simulink model "AutopilotControlSystem"  (R2019b)
settings: configuration reference "ctrlConfigSet" (kept outside this file)
undefined symbols (not defined in the file): ap, DiscIntNeverNeededParam, Earth, env, sensors, uav, WGS84
libraries: mbdriLib x74, simulink x12, aerolibtransform2 x5, simulink_need_slupdate x1, aerolibconvert2 x1
(part 1 of 3)
settings Model: ParamWorkspaceSource=ReferencedWorkspace  Creator=mlizarra  LastModifiedBy=ben
settings ConfigSetRef: SourceName=ctrlConfigSet  SourceLocation=Base Workspace

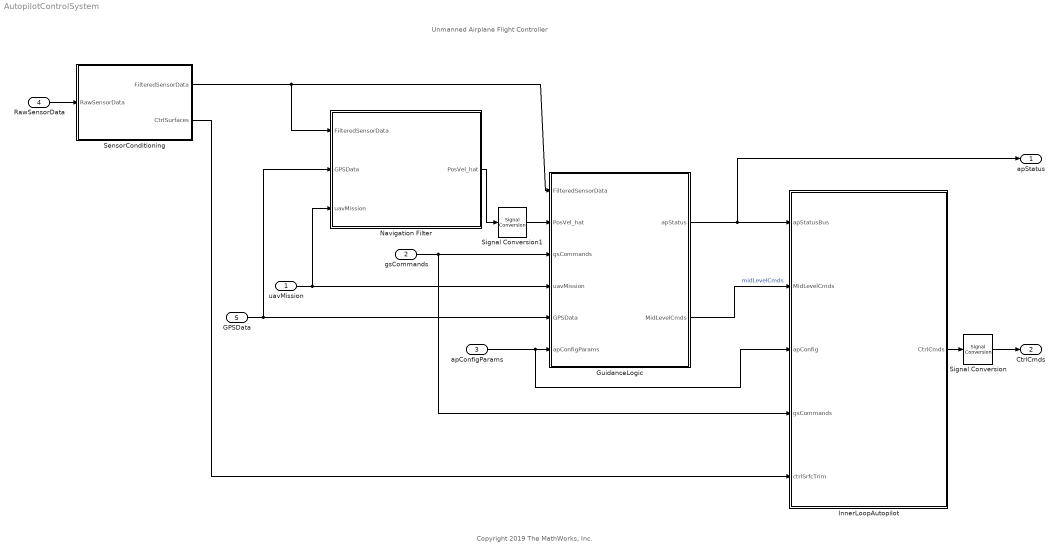
== system AutopilotControlSystem ==
  note: Copyright 2019 The MathWorks, Inc.
  note: Unmanned Airplane Flight Controller
  uavMission : Inport  OutDataTypeStr=Bus: waypoint  PortDimensions=10  SampleTime=[0.01,0]  BusOutputAsStruct=on
  gsCommands : Inport  Port=2  OutDataTypeStr=Bus: gsCommandsBus  PortDimensions=1  SampleTime=[0.01,0]  BusOutputAsStruct=on
  apConfigParams : Inport  Port=3  OutDataTypeStr=Bus: apConfigParamsBus  PortDimensions=1  SampleTime=[0.01,0]  BusOutputAsStruct=on
  RawSensorData : Inport  Port=4  OutDataTypeStr=Bus: rawSensorDataBus  PortDimensions=1  SampleTime=[0.01,0]  BusOutputAsStruct=on
  GPSData : Inport  Port=5  OutDataTypeStr=Bus: gpsReading  PortDimensions=1  SampleTime=[0.01,0]  BusOutputAsStruct=on
  GuidanceLogic : Subsystem  Variant=on  VariantControl=Variant1
  InnerLoopAutopilot : Subsystem  TreatAsAtomicUnit=on
  Navigation Filter : Subsystem  TreatAsAtomicUnit=on
  SensorConditioning : Subsystem  TreatAsAtomicUnit=on
  Signal Conversion : SignalConversion  ConversionOutput=Nonvirtual bus  OutDataTypeStr=Bus: ctrlCmdsBus  OverrideOpt=off
  Signal Conversion1 : SignalConversion  ConversionOutput=Nonvirtual bus  OutDataTypeStr=Bus: PosVel_hat  OverrideOpt=off
  apStatus : Outport  OutDataTypeStr=Bus: apStatusBus  PortDimensions=1  SampleTime=[0.01,0]  VectorParamsAs1DForOutWhenUnconnected=off  BusOutputAsStruct=on
  CtrlCmds : Outport  Port=2  OutDataTypeStr=Bus: ctrlCmdsBus  SampleTime=[0.01,0]  VectorParamsAs1DForOutWhenUnconnected=off  BusOutputAsStruct=on
  wires:
  gsCommands/1 -> GuidanceLogic/3("gsCommands "), InnerLoopAutopilot/4(gsCommands)
  uavMission/1 -> Navigation Filter/3(uavMission), GuidanceLogic/4("uavMission ")
  GuidanceLogic/2(" MidLevelCmds") -> InnerLoopAutopilot/2(MidLevelCmds)  "midLevelCmds"
  Navigation Filter/1(PosVel_hat) -> Signal Conversion1/1
  GPSData/1 -> Navigation Filter/2(GPSData), GuidanceLogic/5("GPSData ")
  SensorConditioning/2(CtrlSurfaces) -> InnerLoopAutopilot/5(ctrlSrfcTrim)
  SensorConditioning/1(FilteredSensorData) -> Navigation Filter/1(FilteredSensorData), GuidanceLogic/1("FilteredSensorData ")
  GuidanceLogic/1(" apStatus") -> InnerLoopAutopilot/1(apStatusBus), apStatus/1
  apConfigParams/1 -> InnerLoopAutopilot/3(apConfig), GuidanceLogic/6("apConfigParams ")
  RawSensorData/1 -> SensorConditioning/1(RawSensorData)
  InnerLoopAutopilot/1(CtrlCmds) -> Signal Conversion/1
  Signal Conversion/1 -> CtrlCmds/1
  Signal Conversion1/1 -> GuidanceLogic/2("PosVel_hat ")

== system AutopilotControlSystem/GuidanceLogic ==
  "FilteredSensorData " : Inport
  "PosVel_hat " : Inport  Port=2
  "gsCommands " : Inport  Port=3
  "uavMission " : Inport  Port=4
  "GPSData " : Inport  Port=5
  "apConfigParams " : Inport  Port=6
  GuidanceLogic_Simulink : Subsystem  TreatAsAtomicUnit=on  VariantControl=useSLguidance
  GuidanceLogic_Stateflow : Subsystem  TreatAsAtomicUnit=on  VariantControl=useSFguidance
  " apStatus" : Outport  VectorParamsAs1DForOutWhenUnconnected=off
  " MidLevelCmds" : Outport  Port=2  VectorParamsAs1DForOutWhenUnconnected=off

== system AutopilotControlSystem/InnerLoopAutopilot ==
  apStatusBus : Inport  OutDataTypeStr=Bus: apStatusBus
  MidLevelCmds : Inport  Port=2
  apConfig : Inport  Port=3  OutDataTypeStr=Bus: apConfigParamsBus
  gsCommands : Inport  Port=4
  ctrlSrfcTrim : Inport  Port=5
  FLapCmd : Constant  Value=0  OutDataTypeStr=single  SampleTime=ap.apSampleTime
      settings: AttributesFormatString=%<Value>
  Latch Trim Conditions : Subsystem
  Lateral Channel : Subsystem  TreatAsAtomicUnit=on
  Longitudinal Channel : Subsystem  TreatAsAtomicUnit=on
  Out Bus Element : Outport  VectorParamsAs1DForOutWhenUnconnected=off  PortName=CtrlCmds  Element=elevatorCmd
  Out Bus Element1 : Outport  VectorParamsAs1DForOutWhenUnconnected=off  PortName=CtrlCmds  Element=throttleCmd
  Out Bus Element2 : Outport  VectorParamsAs1DForOutWhenUnconnected=off  PortName=CtrlCmds  Element=aileronCmd
  Out Bus Element3 : Outport  VectorParamsAs1DForOutWhenUnconnected=off  PortName=CtrlCmds  Element=rudderCmd
  Out Bus Element4 : Outport  VectorParamsAs1DForOutWhenUnconnected=off  PortName=CtrlCmds  Element=flapCmd
  wires:
  gsCommands/1 -> Latch Trim Conditions/2(gsCommands), Lateral Channel/5(gsCommands), Longitudinal Channel/5(gsCommands)
  Latch Trim Conditions/1(CtrlSrfcTrim) -> Lateral Channel/4(ctrlSrfcTrim), Longitudinal Channel/4(ctrlSrfcTrim)
  ctrlSrfcTrim/1 -> Latch Trim Conditions/1(ctrlSurfaces)
  apConfig/1 -> Lateral Channel/3(apConfigBus), Longitudinal Channel/3(apConfigBus)
  FLapCmd/1 -> Out Bus Element4/1
  Lateral Channel/2(dR) -> Out Bus Element3/1
  Lateral Channel/1(dA) -> Out Bus Element2/1
  Longitudinal Channel/2(dT) -> Out Bus Element1/1
  Longitudinal Channel/1(dE) -> Out Bus Element/1
  apStatusBus/1 -> Lateral Channel/2(apStatusBus), Longitudinal Channel/2(apStatusBus)
  MidLevelCmds/1 -> Lateral Channel/1(midLevelCmds), Longitudinal Channel/1(midLevelCmds)

== system AutopilotControlSystem/Navigation Filter ==
  In Bus Element5 : Inport  PortName=FilteredSensorData  Element=Euler
  In Bus Element6 : Inport  PortName=FilteredSensorData  Element=Ab
  In Bus Element7 : Inport  PortName=FilteredSensorData  Element=baro
  In Bus Element : Inport  Port=2  PortName=GPSData  Element=gps_fix
  In Bus Element1 : Inport  Port=2  PortName=GPSData  Element=gps_latLon
  In Bus Element2 : Inport  Port=2  PortName=GPSData  Element=gps_h
  In Bus Element3 : Inport  Port=2  PortName=GPSData  Element=gps_cog
  In Bus Element4 : Inport  Port=2  PortName=GPSData  Element=gps_sog
  uavMission : Inport  Port=3  OutDataTypeStr=Bus: waypoint
  Baro Altimeter : Subsystem
  Bus Selector1 : BusSelector  OutputSignals=wpPos
  Compare To Constant : simulink/Logic and Bit Operations/Compare To Constant  relop=>=  const=3  OutDataTypeStr=boolean
  GPS Update : Subsystem  mask{T=ap.apSampleTime}
      mask prompts: T "Sample Time"
  Get Vn Ve : Subsystem
  LLA to Flat Earth : Subsystem
  Position&Velocity Filter : Subsystem
  RL2B : mbdriLib/Coordinates/RL2B  SystemSampleTime=-1  Latency=0  AutoFrameSizeCalculation=off
      settings: SourceProductName=Robotics System Toolbox  SourceProductBaseCode=RO
  Selector : Selector  InputPortWidth=10  IndexOptions=Index vector (dialog)  Indices=[1]  OutputSizes=1
  get Height : Selector  InputPortWidth=3  IndexOptions=Index vector (dialog)  Indices=[3]  OutputSizes=1
  Out Bus Element : Outport  VectorParamsAs1DForOutWhenUnconnected=off  PortName=PosVel_hat  Element=Ve_hat
  Out Bus Element1 : Outport  VectorParamsAs1DForOutWhenUnconnected=off  PortName=PosVel_hat  Element=Xe_hat
  Out Bus Element2 : Outport  VectorParamsAs1DForOutWhenUnconnected=off  PortName=PosVel_hat  Element=Ab_bias_hat
  wires:
  LLA to Flat Earth/1(Xe) -> Position&Velocity Filter/2(Xe), GPS Update/1(Xe)
  get Height/1 -> Position&Velocity Filter/9(Base Height)
  In Bus Element6/1 -> Position&Velocity Filter/7(A_sens)
  RL2B/1 -> Position&Velocity Filter/6(RLT2B)
  In Bus Element5/1 -> RL2B/1
  In Bus Element7/1 -> Baro Altimeter/1(Static (Pa))
  Baro Altimeter/1(Altitude) -> Position&Velocity Filter/8(BaroAlt)
  Get Vn Ve/2(Veast) -> Position&Velocity Filter/4(Veast)
  Get Vn Ve/1(Vnorth) -> Position&Velocity Filter/3(Vnorth)
  GPS Update/1(Update?) -> Position&Velocity Filter/1(NewGPS)
  Selector/1 -> Bus Selector1/1
  uavMission/1 -> Selector/1
  Bus Selector1/1 -> LLA to Flat Earth/5(initPos), get Height/1  "<wpPos>"
  In Bus Element4/1 -> LLA to Flat Earth/4(SOG)
  In Bus Element3/1 -> LLA to Flat Earth/3(COG)
  In Bus Element2/1 -> LLA to Flat Earth/2(h)
  In Bus Element1/1 -> LLA to Flat Earth/1(latLon)
  Compare To Constant/1 -> LLA to Flat Earth/Enable
  In Bus Element/1 -> Compare To Constant/1
  Position&Velocity Filter/2(Xe_hat) -> Out Bus Element1/1
  Position&Velocity Filter/1(Ve_hat) -> Out Bus Element/1
  Position&Velocity Filter/3(acc_bias) -> Out Bus Element2/1
  LLA to Flat Earth/2(COG_out) -> Get Vn Ve/1(COG)
  LLA to Flat Earth/3(SOG_out) -> Get Vn Ve/2(SOG), Position&Velocity Filter/5(SOG)

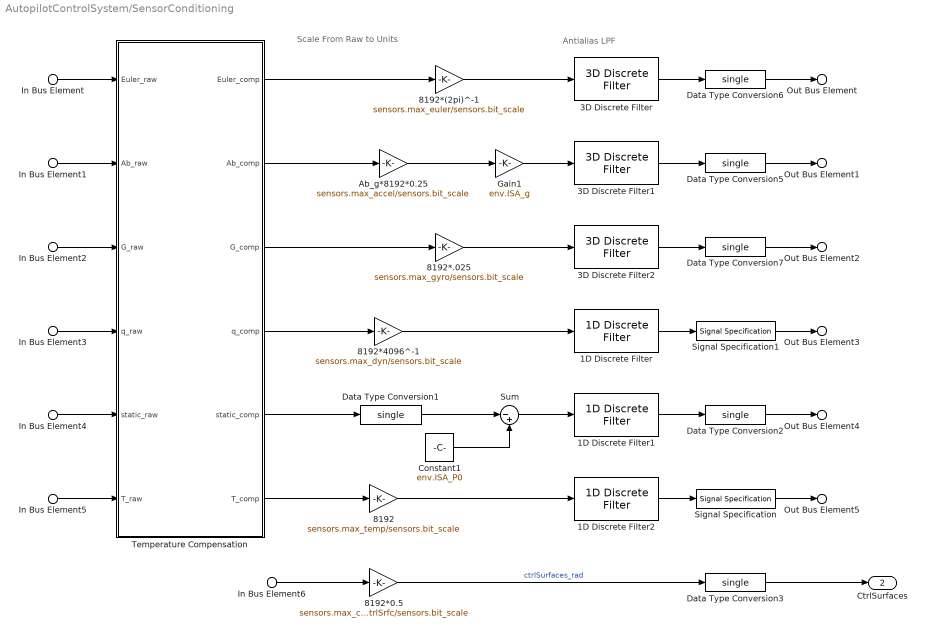
== system AutopilotControlSystem/SensorConditioning ==
  note: Antialias LPF
  note: Scale From Raw to Units
  In Bus Element : Inport  PortName=RawSensorData  Element=Euler_raw
  In Bus Element1 : Inport  PortName=RawSensorData  Element=Ab_raw
  In Bus Element2 : Inport  PortName=RawSensorData  Element=G_raw
  In Bus Element3 : Inport  PortName=RawSensorData  Element=q_raw
  In Bus Element4 : Inport  PortName=RawSensorData  Element=static_raw
  In Bus Element5 : Inport  PortName=RawSensorData  Element=T_raw
  In Bus Element6 : Inport  PortName=RawSensorData  Element=ctrlSurface_PWM
  1D Discrete Filter : mbdriLib/Filtering/1D Discrete Filter  bw=sensors.antialiasBW  TSample=ap.apSampleTime
      settings: AttributesFormatString=Fc = 40  SourceProductName=Robotics System Toolbox  SourceProductBaseCode=RO
  1D Discrete Filter1 : mbdriLib/Filtering/1D Discrete Filter  bw=sensors.antialiasBW  TSample=ap.apSampleTime
      settings: AttributesFormatString=Fc = 40  SourceProductName=Robotics System Toolbox  SourceProductBaseCode=RO
  1D Discrete Filter2 : mbdriLib/Filtering/1D Discrete Filter  bw=sensors.antialiasBW  TSample=ap.apSampleTime
      settings: AttributesFormatString=Fc = 40  SourceProductName=Robotics System Toolbox  SourceProductBaseCode=RO
  3D Discrete Filter : mbdriLib/Filtering/3D Discrete Filter  bw=sensors.antialiasBW  TSample=ap.apSampleTime
      settings: AttributesFormatString=Fc = 40  SourceProductName=Robotics System Toolbox  SourceProductBaseCode=RO
  3D Discrete Filter1 : mbdriLib/Filtering/3D Discrete Filter  bw=sensors.antialiasBW  TSample=ap.apSampleTime
      settings: AttributesFormatString=Fc = 40  SourceProductName=Robotics System Toolbox  SourceProductBaseCode=RO
  3D Discrete Filter2 : mbdriLib/Filtering/3D Discrete Filter  bw=sensors.antialiasBW  TSample=ap.apSampleTime
      settings: AttributesFormatString=Fc = 40  SourceProductName=Robotics System Toolbox  SourceProductBaseCode=RO
  8192 : Gain  Description=8192/1  Gain=sensors.max_temp/sensors.bit_scale  OutDataTypeStr=single
      settings: AttributesFormatString=%<Gain>
  8192*(2pi)^-1 : Gain  Gain=sensors.max_euler/sensors.bit_scale  OutDataTypeStr=single
      settings: AttributesFormatString=%<Gain>
  8192*.025 : Gain  Gain=sensors.max_gyro/sensors.bit_scale  OutDataTypeStr=single
      settings: AttributesFormatString=%<Gain>
  8192*0.5 : Gain  Gain=sensors.max_ctrlSrfc/sensors.bit_scale  OutDataTypeStr=single
      settings: AttributesFormatString=%<Gain>
  8192*4096^-1 : Gain  Gain=sensors.max_dyn/sensors.bit_scale  OutDataTypeStr=single
      settings: AttributesFormatString=%<Gain>
  Ab_g*8192*0.25 : Gain  Gain=sensors.max_accel/sensors.bit_scale  OutDataTypeStr=single
      settings: AttributesFormatString=%<Gain>
  Constant1 : Constant  Value=env.ISA_P0
      settings: AttributesFormatString=%<Value>
  Data Type Conversion{1..3,5..7} (6 alike) : DataTypeConversion  OutDataTypeStr=single
  Gain1 : Gain  Gain=env.ISA_g  OutDataTypeStr=single
      settings: AttributesFormatString=%<Gain>
  Signal Specification : SignalSpecification  OutDataTypeStr=single  Unit=K
  Signal Specification1 : SignalSpecification  OutDataTypeStr=single  Unit=Pa
  Sum : Sum  Inputs=|-+
  Temperature Compensation : Subsystem
  Out Bus Element : Outport  VectorParamsAs1DForOutWhenUnconnected=off  PortName=FilteredSensorData  Element=Euler
  Out Bus Element1 : Outport  VectorParamsAs1DForOutWhenUnconnected=off  PortName=FilteredSensorData  Element=Ab
  Out Bus Element2 : Outport  VectorParamsAs1DForOutWhenUnconnected=off  PortName=FilteredSensorData  Element=G
  Out Bus Element3 : Outport  VectorParamsAs1DForOutWhenUnconnected=off  PortName=FilteredSensorData  Element=q
  Out Bus Element4 : Outport  VectorParamsAs1DForOutWhenUnconnected=off  PortName=FilteredSensorData  Element=baro
  Out Bus Element5 : Outport  VectorParamsAs1DForOutWhenUnconnected=off  PortName=FilteredSensorData  Element=T
  CtrlSurfaces : Outport  Port=2  VectorParamsAs1DForOutWhenUnconnected=off
  wires:
  8192*0.5/1 -> Data Type Conversion3/1  "ctrlSurfaces_rad"
  In Bus Element6/1 -> 8192*0.5/1
  Data Type Conversion3/1 -> CtrlSurfaces/1
  1D Discrete Filter2/1 -> Signal Specification/1
  Data Type Conversion2/1 -> Out Bus Element4/1
  1D Discrete Filter1/1 -> Data Type Conversion2/1
  1D Discrete Filter/1 -> Signal Specification1/1
  3D Discrete Filter2/1 -> Data Type Conversion7/1
  3D Discrete Filter1/1 -> Data Type Conversion5/1
  3D Discrete Filter/1 -> Data Type Conversion6/1
  Data Type Conversion1/1 -> Sum/1
  Gain1/1 -> 3D Discrete Filter1/1
  Data Type Conversion6/1 -> Out Bus Element/1
  Data Type Conversion5/1 -> Out Bus Element1/1
  Data Type Conversion7/1 -> Out Bus Element2/1
  Signal Specification1/1 -> Out Bus Element3/1
  Sum/1 -> 1D Discrete Filter1/1
  Signal Specification/1 -> Out Bus Element5/1
  Constant1/1 -> Sum/2
  8192/1 -> 1D Discrete Filter2/1
  8192*4096^-1/1 -> 1D Discrete Filter/1
  8192*.025/1 -> 3D Discrete Filter2/1
  8192*(2pi)^-1/1 -> 3D Discrete Filter/1
  Ab_g*8192*0.25/1 -> Gain1/1
  In Bus Element/1 -> Temperature Compensation/1(Euler_raw)
  In Bus Element1/1 -> Temperature Compensation/2(Ab_raw)
  In Bus Element2/1 -> Temperature Compensation/3(G_raw)
  In Bus Element3/1 -> Temperature Compensation/4(q_raw)
  In Bus Element4/1 -> Temperature Compensation/5(static_raw)
  In Bus Element5/1 -> Temperature Compensation/6(T_raw)
  Temperature Compensation/1(Euler_comp) -> 8192*(2pi)^-1/1
  Temperature Compensation/2(Ab_comp) -> Ab_g*8192*0.25/1
  Temperature Compensation/3(G_comp) -> 8192*.025/1
  Temperature Compensation/4(q_comp) -> 8192*4096^-1/1
  Temperature Compensation/5(static_comp) -> Data Type Conversion1/1
  Temperature Compensation/6(T_comp) -> 8192/1

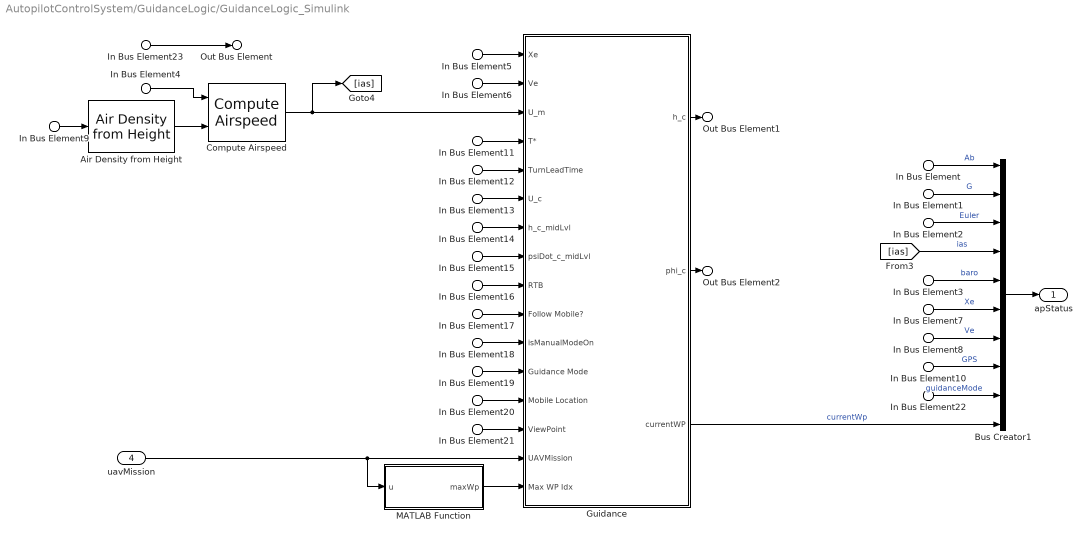
== system AutopilotControlSystem/GuidanceLogic/GuidanceLogic_Simulink ==
  In Bus Element : Inport  PortName=FilteredSensorData  Element=Ab
  In Bus Element1 : Inport  PortName=FilteredSensorData  Element=G
  In Bus Element2 : Inport  PortName=FilteredSensorData  Element=Euler
  In Bus Element3 : Inport  PortName=FilteredSensorData  Element=baro
  In Bus Element4 : Inport  PortName=FilteredSensorData  Element=q
  In Bus Element5 : Inport  Port=2  PortName=PosVel_hat  Element=Xe_hat
  In Bus Element7 : Inport  Port=2  PortName=PosVel_hat  Element=Xe_hat
  In Bus Element6 : Inport  Port=2  PortName=PosVel_hat  Element=Ve_hat
  In Bus Element8 : Inport  Port=2  PortName=PosVel_hat  Element=Ve_hat
  In Bus Element13 : Inport  Port=3  PortName=gsCommands  Element=U_c
  In Bus Element23 : Inport  Port=3  PortName=gsCommands  Element=U_c
  In Bus Element14 : Inport  Port=3  PortName=gsCommands  Element=h_c_midLevel
  In Bus Element15 : Inport  Port=3  PortName=gsCommands  Element=psiDot_c_midLevel
  In Bus Element16 : Inport  Port=3  PortName=gsCommands  Element=RTB
  In Bus Element17 : Inport  Port=3  PortName=gsCommands  Element=followMobile
  In Bus Element18 : Inport  Port=3  PortName=gsCommands  Element=isManualModeOn
  In Bus Element19 : Inport  Port=3  PortName=gsCommands  Element=guidanceMode
  In Bus Element22 : Inport  Port=3  PortName=gsCommands  Element=guidanceMode
  In Bus Element20 : Inport  Port=3  PortName=gsCommands  Element=MobileLocation
  In Bus Element21 : Inport  Port=3  PortName=gsCommands  Element=viewPointIdx
  uavMission : Inport  Port=4
  In Bus Element10 : Inport  Port=5  PortName=GPSData
  In Bus Element9 : Inport  Port=5  PortName=GPSData  Element=gps_h
  In Bus Element11 : Inport  Port=6  PortName=apConfigParams  Element=T_star
  In Bus Element12 : Inport  Port=6  PortName=apConfigParams  Element=turnLead
  Air Density from Height : mbdriLib/Air Utilities/Air Density from Height  SystemSampleTime=-1  Latency=0  AutoFrameSizeCalculation=off
      settings: SourceProductName=Robotics System Toolbox  SourceProductBaseCode=RO
  Bus Creator1 : BusCreator  Inputs=10  OutDataTypeStr=Bus: apStatusBus  NonVirtualBus=on
  Compute Airspeed : mbdriLib/Air Utilities/Compute Airspeed  SystemSampleTime=-1  Latency=0  AutoFrameSizeCalculation=off
      settings: SourceProductName=Robotics System Toolbox  SourceProductBaseCode=RO
  Guidance : Subsystem  TreatAsAtomicUnit=on
  MATLAB Function : MATLAB Function  TreatAsAtomicUnit=on
  apStatus : Outport  VectorParamsAs1DForOutWhenUnconnected=off
  Out Bus Element : Outport  Port=2  VectorParamsAs1DForOutWhenUnconnected=off  PortName=MidLevelCmds  Element=U_c
  Out Bus Element1 : Outport  Port=2  VectorParamsAs1DForOutWhenUnconnected=off  PortName=MidLevelCmds  Element=h_c
  Out Bus Element2 : Outport  Port=2  VectorParamsAs1DForOutWhenUnconnected=off  PortName=MidLevelCmds  Element=phi_c
  wires:
  Guidance/3(currentWP) -> Bus Creator1/10  "currentWp"
  In Bus Element22/1 -> Bus Creator1/9  "guidanceMode"
  In Bus Element10/1 -> Bus Creator1/8  "GPS"
  In Bus Element8/1 -> Bus Creator1/7  "Ve"
  In Bus Element7/1 -> Bus Creator1/6  "Xe"
  In Bus Element3/1 -> Bus Creator1/5  "baro"
  [ias] -> Bus Creator1/4  "ias"
  In Bus Element2/1 -> Bus Creator1/3  "Euler"
  In Bus Element1/1 -> Bus Creator1/2  "G"
  In Bus Element/1 -> Bus Creator1/1  "Ab"
  Bus Creator1/1 -> apStatus/1
  Guidance/2(phi_c) -> Out Bus Element2/1
  Guidance/1(h_c) -> Out Bus Element1/1
  In Bus Element9/1 -> Air Density from Height/1
  In Bus Element12/1 -> Guidance/5(TurnLeadTime)
  In Bus Element11/1 -> Guidance/4("T* ")
  MATLAB Function/1(maxWp) -> Guidance/16(Max WP Idx)
  In Bus Element4/1 -> Compute Airspeed/1
  Compute Airspeed/1 -> Guidance/3(U_m), [ias]
  Air Density from Height/1 -> Compute Airspeed/2
  In Bus Element21/1 -> Guidance/14(ViewPoint)
  In Bus Element20/1 -> Guidance/13(Mobile Location)
  In Bus Element19/1 -> Guidance/12(Guidance Mode)
  In Bus Element18/1 -> Guidance/11(isManualModeOn)
  In Bus Element17/1 -> Guidance/10(Follow Mobile?)
  In Bus Element16/1 -> Guidance/9(RTB)
  In Bus Element15/1 -> Guidance/8(psiDot_c_midLvl)
  In Bus Element14/1 -> Guidance/7(h_c_midLvl)
  In Bus Element13/1 -> Guidance/6(U_c)
  In Bus Element6/1 -> Guidance/2(Ve)
  In Bus Element5/1 -> Guidance/1(Xe)
  uavMission/1 -> Guidance/15(UAVMission), MATLAB Function/1(u)
  In Bus Element23/1 -> Out Bus Element/1

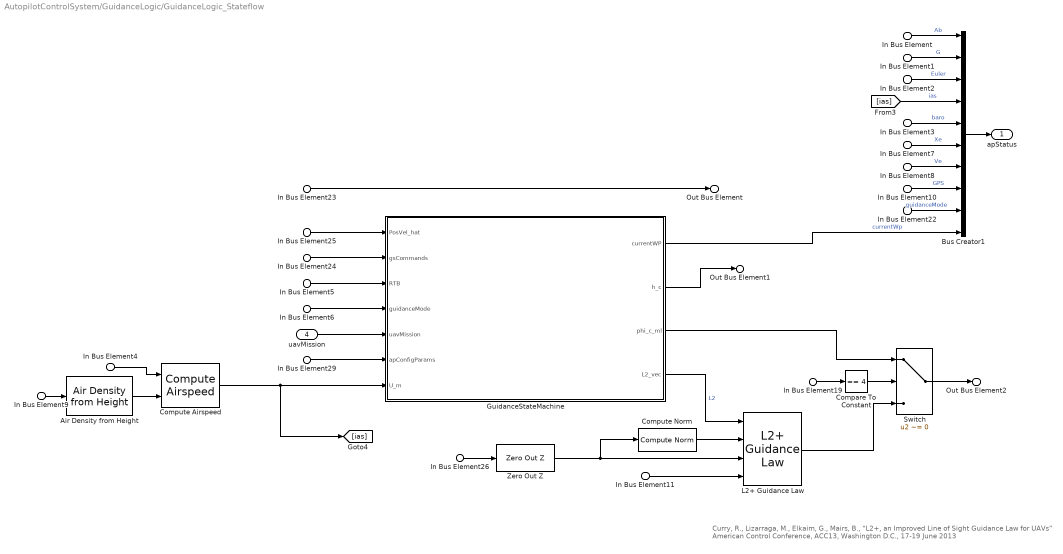
== system AutopilotControlSystem/GuidanceLogic/GuidanceLogic_Stateflow ==
  note: Curry, R., Lizarraga, M., Elkaim, G., Mairs, B., “L2+, an Improved Line of Sight Guidance Law for UAVs”
      | American Control Conference, ACC13, Washington D.C., 17-19 June 2013
  In Bus Element : Inport  PortName=FilteredSensorData  Element=Ab
  In Bus Element1 : Inport  PortName=FilteredSensorData  Element=G
  In Bus Element2 : Inport  PortName=FilteredSensorData  Element=Euler
  In Bus Element3 : Inport  PortName=FilteredSensorData  Element=baro
  In Bus Element4 : Inport  PortName=FilteredSensorData  Element=q
  In Bus Element25 : Inport  Port=2  PortName=PosVel_hat
  In Bus Element7 : Inport  Port=2  PortName=PosVel_hat  Element=Xe_hat
  In Bus Element8 : Inport  Port=2  PortName=PosVel_hat  Element=Ve_hat
  In Bus Element26 : Inport  Port=2  PortName=PosVel_hat  Element=Ve_hat
  In Bus Element24 : Inport  Port=3  PortName=gsCommands
  In Bus Element23 : Inport  Port=3  PortName=gsCommands  Element=U_c
  In Bus Element19 : Inport  Port=3  PortName=gsCommands  Element=guidanceMode
  In Bus Element22 : Inport  Port=3  PortName=gsCommands  Element=guidanceMode
  In Bus Element6 : Inport  Port=3  PortName=gsCommands  Element=guidanceMode
  In Bus Element5 : Inport  Port=3  PortName=gsCommands  Element=RTB
  uavMission : Inport  Port=4
  In Bus Element10 : Inport  Port=5  PortName=GPSData
  In Bus Element9 : Inport  Port=5  PortName=GPSData  Element=gps_h
  In Bus Element29 : Inport  Port=6  PortName=apConfigParams
  In Bus Element11 : Inport  Port=6  PortName=apConfigParams  Element=T_star
  " Compute Norm" : mbdriLib/Utilities/ Compute Norm  SystemSampleTime=-1  Latency=0  AutoFrameSizeCalculation=off
      settings: SourceProductName=Robotics System Toolbox  SourceProductBaseCode=RO
  Air Density from Height : mbdriLib/Air Utilities/Air Density from Height  SystemSampleTime=-1  Latency=0  AutoFrameSizeCalculation=off
      settings: SourceProductName=Robotics System Toolbox  SourceProductBaseCode=RO
  Bus Creator1 : BusCreator  Inputs=10  OutDataTypeStr=Bus: apStatusBus  NonVirtualBus=on
  Compare To Constant : simulink/Logic and Bit Operations/Compare To Constant  relop===  const=4  OutDataTypeStr=boolean
  Compute Airspeed : mbdriLib/Air Utilities/Compute Airspeed  SystemSampleTime=-1  Latency=0  AutoFrameSizeCalculation=off
      settings: SourceProductName=Robotics System Toolbox  SourceProductBaseCode=RO
  GuidanceStateMachine : Stateflow chart  TreatAsAtomicUnit=on
  L2+ Guidance Law : mbdriLib/Guidance/L2+ Guidance Law  SystemSampleTime=-1  Latency=0  AutoFrameSizeCalculation=off
      settings: SourceProductName=Robotics System Toolbox  SourceProductBaseCode=RO
  Switch : Switch  Criteria=u2 ~= 0  Threshold=3.1
  Zero Out Z : mbdriLib/Utilities/Zero Out Z  SystemSampleTime=-1  Latency=0  AutoFrameSizeCalculation=off
      settings: SourceProductName=Robotics System Toolbox  SourceProductBaseCode=RO
  apStatus : Outport  VectorParamsAs1DForOutWhenUnconnected=off
  Out Bus Element : Outport  Port=2  VectorParamsAs1DForOutWhenUnconnected=off  PortName=MidLevelCmds  Element=U_c
  Out Bus Element1 : Outport  Port=2  VectorParamsAs1DForOutWhenUnconnected=off  PortName=MidLevelCmds  Element=h_c
  Out Bus Element2 : Outport  Port=2  VectorParamsAs1DForOutWhenUnconnected=off  PortName=MidLevelCmds  Element=phi_c
  wires:
  In Bus Element23/1 -> Out Bus Element/1
  Air Density from Height/1 -> Compute Airspeed/2
  In Bus Element4/1 -> Compute Airspeed/1
  In Bus Element9/1 -> Air Density from Height/1
  Bus Creator1/1 -> apStatus/1
  In Bus Element/1 -> Bus Creator1/1  "Ab"
  In Bus Element1/1 -> Bus Creator1/2  "G"
  In Bus Element2/1 -> Bus Creator1/3  "Euler"
  [ias] -> Bus Creator1/4  "ias"
  In Bus Element3/1 -> Bus Creator1/5  "baro"
  In Bus Element7/1 -> Bus Creator1/6  "Xe"
  In Bus Element8/1 -> Bus Creator1/7  "Ve"
  In Bus Element10/1 -> Bus Creator1/8  "GPS"
  In Bus Element22/1 -> Bus Creator1/9  "guidanceMode"
  In Bus Element24/1 -> GuidanceStateMachine/2(gsCommands)
  uavMission/1 -> GuidanceStateMachine/5(uavMission)
  In Bus Element25/1 -> GuidanceStateMachine/1(PosVel_hat)
  In Bus Element29/1 -> GuidanceStateMachine/6(apConfigParams)
  Compute Airspeed/1 -> GuidanceStateMachine/7(U_m), [ias]
  GuidanceStateMachine/1(currentWP) -> Bus Creator1/10  "currentWp"
  GuidanceStateMachine/2(h_c) -> Out Bus Element1/1
  Switch/1 -> Out Bus Element2/1
  " Compute Norm"/1 -> L2+ Guidance Law/2
  GuidanceStateMachine/4(L2_vec) -> L2+ Guidance Law/1  "L2"
  In Bus Element11/1 -> L2+ Guidance Law/4
  Zero Out Z/1 -> L2+ Guidance Law/3, " Compute Norm"/1
  GuidanceStateMachine/3(phi_c_ml) -> Switch/1
  In Bus Element19/1 -> Compare To Constant/1
  L2+ Guidance Law/1 -> Switch/3
  In Bus Element26/1 -> Zero Out Z/1
  In Bus Element5/1 -> GuidanceStateMachine/3(RTB)
  In Bus Element6/1 -> GuidanceStateMachine/4(guidanceMode)
  Compare To Constant/1 -> Switch/2

== system AutopilotControlSystem/InnerLoopAutopilot/Latch Trim Conditions ==
  ctrlSurfaces : Inport
  In Bus Element : Inport  Port=2  PortName=gsCommands  Element=isManualModeOn
  Compare To Constant : simulink/Logic and Bit Operations/Compare To Constant  relop===  const=1  OutDataTypeStr=boolean
  Latch Control Surfaces Trim from any mode : Subsystem  TreatAsAtomicUnit=on
  CtrlSrfcTrim : Outport  VectorParamsAs1DForOutWhenUnconnected=off
  wires:
  In Bus Element/1 -> Compare To Constant/1
  Latch Control Surfaces Trim from any mode/1(Trim) -> CtrlSrfcTrim/1
  Compare To Constant/1 -> Latch Control Surfaces Trim from any mode/Trigger
  ctrlSurfaces/1 -> Latch Control Surfaces Trim from any mode/1(ctrlSurfaces)

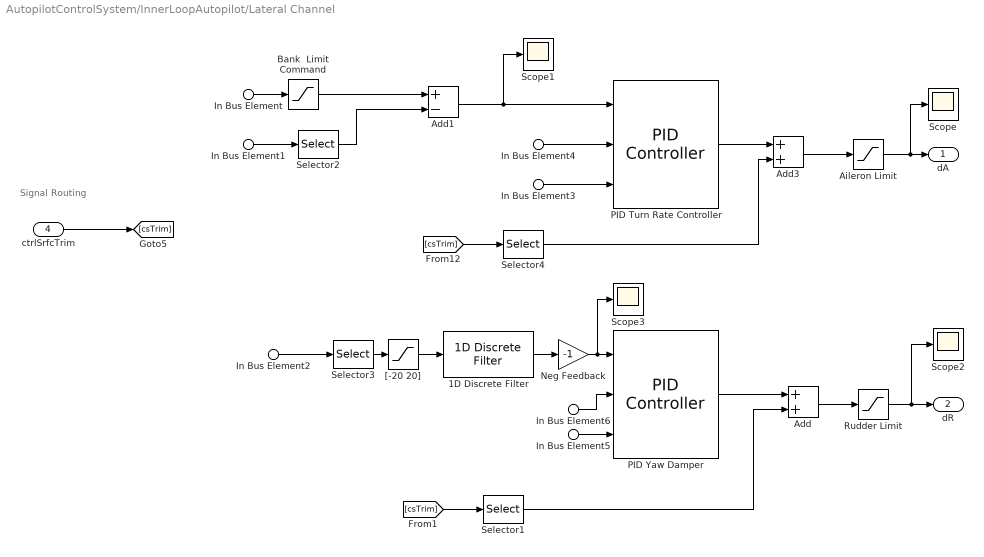
== system AutopilotControlSystem/InnerLoopAutopilot/Lateral Channel ==
  note: Signal Routing
  In Bus Element : Inport  PortName=midLevelCmds  Element=phi_c
  In Bus Element1 : Inport  Port=2  PortName=apStatusBus  Element=Euler
  In Bus Element2 : Inport  Port=2  PortName=apStatusBus  Element=Ab
  In Bus Element3 : Inport  Port=3  PortName=apConfigBus  Element=rollControlPID
  In Bus Element5 : Inport  Port=3  PortName=apConfigBus  Element=yawDamperPID
  ctrlSrfcTrim : Inport  Port=4
  In Bus Element4 : Inport  Port=5  PortName=gsCommands  Element=isManualModeOn
  In Bus Element6 : Inport  Port=5  PortName=gsCommands  Element=isManualModeOn
  1D Discrete Filter : mbdriLib/Filtering/1D Discrete Filter  bw=10  TSample=ap.apSampleTime
      settings: AttributesFormatString=Fc = 10  SourceProductName=Robotics System Toolbox  SourceProductBaseCode=RO
  Add : Sum  OutDataTypeStr=single
  Add1 : Sum  Inputs=+-  OutDataTypeStr=single
  Add3 : Sum  OutDataTypeStr=single
  Aileron Limit : Saturate  UpperLimit=ap.control.daLimit  LowerLimit=-ap.control.daLimit
      settings: AttributesFormatString="[%<LowerLimit>  %<UpperLimit>]"
  Bank  Limit Command : Saturate  UpperLimit=ap.control.phi_cLimit  LowerLimit=-ap.control.phi_cLimit
      settings: AttributesFormatString="[%<LowerLimit>  %<UpperLimit>]"
  Neg Feedback : Gain  Gain=-1  OutDataTypeStr=float('double')
      settings: AttributesFormatString=%<Gain>
  PID Turn Rate Controller : mbdriLib/Control/PID Controller  Tsample=ap.apSampleTime  Ndelay=ap.control.derivativesConstant  upperSaturationLimit=ap.control.daLimit  lowerSaturationLimit=-ap.control.daLimit
      settings: SourceProductName=Robotics System Toolbox  SourceProductBaseCode=RO
  PID Yaw Damper : mbdriLib/Control/PID Controller  Tsample=ap.apSampleTime  Ndelay=ap.control.derivativesConstant  upperSaturationLimit=ap.control.drLimit  lowerSaturationLimit=-ap.control.drLimit
      settings: SourceProductName=Robotics System Toolbox  SourceProductBaseCode=RO
  Rudder Limit : Saturate  UpperLimit=ap.control.drLimit  LowerLimit=-ap.control.drLimit
      settings: AttributesFormatString="[%<LowerLimit>  %<UpperLimit>]"
  Scope{,1..3} (4 alike) : Scope
  Selector1 : Selector  InputPortWidth=5  IndexOptions=Index vector (dialog)  Indices=[3]  OutputSizes=1
  Selector2 : Selector  InputPortWidth=3  IndexOptions=Index vector (dialog)  Indices=[1]  OutputSizes=1
  Selector3 : Selector  InputPortWidth=3  IndexOptions=Index vector (dialog)  Indices=[2]  OutputSizes=1
  Selector4 : Selector  InputPortWidth=5  IndexOptions=Index vector (dialog)  Indices=[2]  OutputSizes=1
  "[-20 20]" : Saturate  UpperLimit=20  LowerLimit=-20
      settings: AttributesFormatString="[%<LowerLimit>  %<UpperLimit>]"
  dA : Outport  VectorParamsAs1DForOutWhenUnconnected=off
  dR : Outport  Port=2  VectorParamsAs1DForOutWhenUnconnected=off
  wires:
  In Bus Element4/1 -> PID Turn Rate Controller/2
  In Bus Element2/1 -> Selector3/1
  Selector3/1 -> "[-20 20]"/1
  In Bus Element6/1 -> PID Yaw Damper/2
  In Bus Element5/1 -> PID Yaw Damper/3
  [csTrim] -> Selector1/1
  [csTrim] -> Selector4/1
  Selector2/1 -> Add1/2
  In Bus Element1/1 -> Selector2/1
  Bank  Limit Command/1 -> Add1/1
  ctrlSrfcTrim/1 -> [csTrim]
  Selector1/1 -> Add/2
  1D Discrete Filter/1 -> Neg Feedback/1
  "[-20 20]"/1 -> 1D Discrete Filter/1
  Selector4/1 -> Add3/2
  Neg Feedback/1 -> Scope3/1, PID Yaw Damper/1
  In Bus Element/1 -> Bank  Limit Command/1
  Add1/1 -> Scope1/1, PID Turn Rate Controller/1
  Aileron Limit/1 -> Scope/1, dA/1
  PID Turn Rate Controller/1 -> Add3/1
  Add3/1 -> Aileron Limit/1
  In Bus Element3/1 -> PID Turn Rate Controller/3
  PID Yaw Damper/1 -> Add/1
  Add/1 -> Rudder Limit/1
  Rudder Limit/1 -> Scope2/1, dR/1

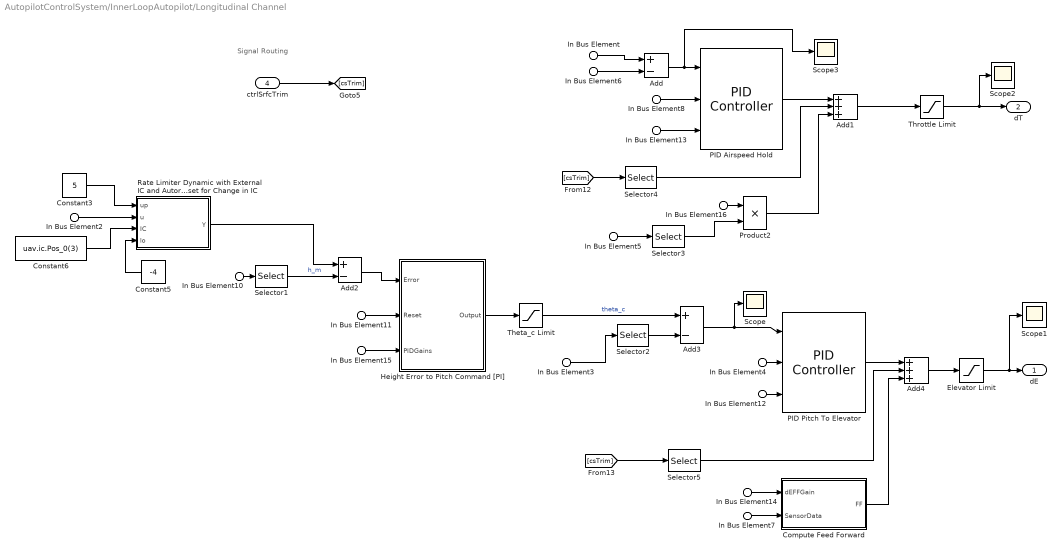
== system AutopilotControlSystem/InnerLoopAutopilot/Longitudinal Channel ==
  note: Signal Routing
  In Bus Element : Inport  PortName=midLevelCmds  Element=U_c
  In Bus Element2 : Inport  PortName=midLevelCmds  Element=h_c
  In Bus Element7 : Inport  Port=2  PortName=apStatusBus
  In Bus Element6 : Inport  Port=2  PortName=apStatusBus  Element=ias
  In Bus Element10 : Inport  Port=2  PortName=apStatusBus  Element=Xe
  In Bus Element3 : Inport  Port=2  PortName=apStatusBus  Element=Euler
  In Bus Element5 : Inport  Port=2  PortName=apStatusBus  Element=Euler
  In Bus Element12 : Inport  Port=3  PortName=apConfigBus  Element=th2dTPID
  In Bus Element13 : Inport  Port=3  PortName=apConfigBus  Element=airspeedHoldPID
  In Bus Element16 : Inport  Port=3  PortName=apConfigBus  Element=dEFeedForward
  In Bus Element15 : Inport  Port=3  PortName=apConfigBus  Element=he2ThPID
  In Bus Element14 : Inport  Port=3  PortName=apConfigBus  Element=dTFeedForward
  ctrlSrfcTrim : Inport  Port=4
  In Bus Element4 : Inport  Port=5  PortName=gsCommands  Element=isManualModeOn
  In Bus Element8 : Inport  Port=5  PortName=gsCommands  Element=isManualModeOn
  In Bus Element11 : Inport  Port=5  PortName=gsCommands  Element=isManualModeOn
  Add : Sum  Inputs=+-
  Add1 : Sum  Inputs=3  OutDataTypeStr=single
  Add2 : Sum  Inputs=+-  OutDataTypeStr=single
  Add3 : Sum  Inputs=+-  OutDataTypeStr=single
  Add4 : Sum  Inputs=3  OutDataTypeStr=single
  Compute Feed Forward : Subsystem
  Constant3 : Constant  Value=5  OutDataTypeStr=single
      settings: AttributesFormatString=%<Value>
  Constant5 : Constant  Value=-4  OutDataTypeStr=single
      settings: AttributesFormatString=%<Value>
  Constant6 : Constant  Value=uav.ic.Pos_0(3)  OutDataTypeStr=single
      settings: AttributesFormatString=%<Value>
  Elevator Limit : Saturate  UpperLimit=ap.control.deLimit  LowerLimit=-ap.control.deLimit
      settings: AttributesFormatString="[%<LowerLimit>  %<UpperLimit>]"
  Height Error to Pitch Command [PI] : Subsystem  mask(PID){Tsample=ap.apSampleTime, Ndelay=ap.control.derivativesConstant, upperSaturationLimit=ap.control.the_cLimit, lowerSaturationLimit=-ap.control.the_cLimit}
      mask prompts: Tsample "Sample Time"; Ndelay "Integer delays for de/dt"; upperSaturationLimit "Upper Saturation Limit"; lowerSaturationLimit "Lower Saturation Limit"
      mask help: PID controller block with anti-windup and saturation limits. Implemented as a discrete forwardl integration which stops integrating when the output is saturated. Derivative is implemented as a numerical derivative with N integer delays to smooth output.
      mask Display:
      | disp('PI')
      | port_label('input',1,'error')
      | port_label('input',3,'gains')
      | port_label('input',2,'reset')
      | port_label('output',1,'output')
  PID Airspeed Hold : mbdriLib/Control/PID Controller  Tsample=ap.apSampleTime  Ndelay=ap.control.derivativesConstant  upperSaturationLimit=ap.control.dtLimit  lowerSaturationLimit=0
      settings: SourceProductName=Robotics System Toolbox  SourceProductBaseCode=RO
  PID Pitch To Elevator : mbdriLib/Control/PID Controller  Tsample=ap.apSampleTime  Ndelay=ap.control.derivativesConstant  upperSaturationLimit=ap.control.deLimit  lowerSaturationLimit=-ap.control.deLimit
      settings: SourceProductName=Robotics System Toolbox  SourceProductBaseCode=RO
  Product2 : Product  RndMeth=Zero
  Rate Limiter Dynamic with External IC and Autoreset for Change in IC : Subsystem
      mask Display:
      | plot([0.15 0.95],[.5 .5],[.5 .5],[0.05 0.95],0.05+0.9*[.2 .8],0.05+0.9*[0 1]);
      | port_label('output',1,'Y');
      | port_label('input',1,'up');
      | port_label('input',2,'u');
      | port_label('input',3,'IC');
      | port_label('input',4,'Lo');
  Scope{,1..3} (4 alike) : Scope
  Selector1 : Selector  InputPortWidth=3  IndexOptions=Index vector (dialog)  Indices=[3]  OutputSizes=1
  Selector2 : Selector  InputPortWidth=3  IndexOptions=Index vector (dialog)  Indices=[2]  OutputSizes=1
  Selector3 : Selector  InputPortWidth=3  IndexOptions=Index vector (dialog)  Indices=[2]  OutputSizes=1
  Selector4 : Selector  InputPortWidth=5  IndexOptions=Index vector (dialog)  Indices=[1]  OutputSizes=1
  Selector5 : Selector  InputPortWidth=5  IndexOptions=Index vector (dialog)  Indices=[5]  OutputSizes=1
  Theta_c Limit : Saturate  UpperLimit=ap.control.the_cLimit  LowerLimit=-ap.control.the_cLimit  SampleTime=ap.apSampleTime
      settings: AttributesFormatString="[%<LowerLimit>  %<UpperLimit>]"
  Throttle Limit : Saturate  UpperLimit=ap.control.dtLimit  LowerLimit=0
      settings: AttributesFormatString="[%<LowerLimit>  %<UpperLimit>]"
  dE : Outport  VectorParamsAs1DForOutWhenUnconnected=off
  dT : Outport  Port=2  VectorParamsAs1DForOutWhenUnconnected=off
  wires:
  Selector5/1 -> Add4/2
  [csTrim] -> Selector5/1
  In Bus Element4/1 -> PID Pitch To Elevator/2
  In Bus Element8/1 -> PID Airspeed Hold/2
  Add4/1 -> Elevator Limit/1
  Elevator Limit/1 -> Scope1/1, dE/1
  Throttle Limit/1 -> Scope2/1, dT/1
  Selector4/1 -> Add1/2
  [csTrim] -> Selector4/1
  ctrlSrfcTrim/1 -> [csTrim]
  In Bus Element5/1 -> Selector3/1
  In Bus Element14/1 -> Compute Feed Forward/1(dEFFGain)
  In Bus Element16/1 -> Product2/1
  Product2/1 -> Add1/3
  Selector3/1 -> Product2/2
  In Bus Element12/1 -> PID Pitch To Elevator/3
  In Bus Element3/1 -> Selector2/1
  Selector2/1 -> Add3/2
  In Bus Element7/1 -> Compute Feed Forward/2(SensorData)
  In Bus Element10/1 -> Selector1/1
  In Bus Element/1 -> Add/1
  Add1/1 -> Throttle Limit/1
  Constant6/1 -> Rate Limiter Dynamic with External IC and Autoreset for Change in IC/3(IC)
  Constant5/1 -> Rate Limiter Dynamic with External IC and Autoreset for Change in IC/4(lo)
  Constant3/1 -> Rate Limiter Dynamic with External IC and Autoreset for Change in IC/1(up)
  In Bus Element15/1 -> Height Error to Pitch Command [PI]/3(PIDGains)
  In Bus Element13/1 -> PID Airspeed Hold/3
  In Bus Element6/1 -> Add/2
  Compute Feed Forward/1(FF) -> Add4/3
  Height Error to Pitch Command [PI]/1(Output) -> Theta_c Limit/1
  Theta_c Limit/1 -> Add3/1  "theta_c"
  Add3/1 -> Scope/1, PID Pitch To Elevator/1
  PID Pitch To Elevator/1 -> Add4/1
  In Bus Element11/1 -> Height Error to Pitch Command [PI]/2(Reset)
  Selector1/1 -> Add2/2  "h_m"
  Add2/1 -> Height Error to Pitch Command [PI]/1(Error)
  PID Airspeed Hold/1 -> Add1/1
  Add/1 -> Scope3/1, PID Airspeed Hold/1
  In Bus Element2/1 -> Rate Limiter Dynamic with External IC and Autoreset for Change in IC/2(u)
  Rate Limiter Dynamic with External IC and Autoreset for Change in IC/1(Y) -> Add2/1

== system AutopilotControlSystem/Navigation Filter/Baro Altimeter ==
  Static (Pa) : Inport
  Constant : Constant  Value=101325
      settings: AttributesFormatString=%<Value>
  Constant1 : Constant  Value=-8.31432
      settings: AttributesFormatString=%<Value>
  Constant2 : Constant  Value=288.15
      settings: AttributesFormatString=%<Value>
  Constant3 : Constant  Value=0.0289644
      settings: AttributesFormatString=%<Value>
  Constant4 : Constant  Value=env.ISA_g
      settings: AttributesFormatString=%<Value>
  Divide : Product  Inputs=*/
  Math Function : Math  Operator=log  SaturateOnIntegerOverflow=on
  Product : Product  Inputs=***//
  "[80k - 120k]" : Saturate  UpperLimit=160000  LowerLimit=80000
      settings: AttributesFormatString="[%<LowerLimit>  %<UpperLimit>]"
  Altitude : Outport  VectorParamsAs1DForOutWhenUnconnected=off
  wires:
  Product/1 -> Altitude/1
  Constant4/1 -> Product/5
  Constant3/1 -> Product/4
  Constant2/1 -> Product/3
  Constant1/1 -> Product/2
  Math Function/1 -> Product/1
  Divide/1 -> Math Function/1
  "[80k - 120k]"/1 -> Divide/1
  Constant/1 -> Divide/2
  Static (Pa)/1 -> "[80k - 120k]"/1

== system AutopilotControlSystem/Navigation Filter/GPS Update ==
  note: If any of the coordinates have changed, set output to 1
  Xe : Inport
  Detect Change : simulink/Logic and Bit Operations/Detect Change  vinit=0  OutDataTypeStr=boolean
  Logical Operator : Logic  Operator=OR  Inputs=1  AllPortsSameDT=off  OutDataTypeStr=boolean
  Update? : Outport  VectorParamsAs1DForOutWhenUnconnected=off
  wires:
  Xe/1 -> Detect Change/1
  Detect Change/1 -> Logical Operator/1
  Logical Operator/1 -> Update?/1

== system AutopilotControlSystem/Navigation Filter/Get Vn Ve ==
  COG : Inport
  SOG : Inport  Port=2
  Angle Conversion : aerolibconvert2/Angle Conversion  IU=deg  OU=rad
  Product : Product  RndMeth=Zero
  Product1 : Product  RndMeth=Zero
  Subsystem5 : Subsystem
  Vnorth : Outport  Unit=m/s  VectorParamsAs1DForOutWhenUnconnected=off
  Veast : Outport  Port=2  Unit=m/s  VectorParamsAs1DForOutWhenUnconnected=off
  wires:
  Product1/1 -> Vnorth/1
  Product/1 -> Veast/1
  SOG/1 -> Product1/1, Product/2
  Angle Conversion/1 -> Subsystem5/1(u)
  Subsystem5/1(sin(u)) -> Product/1
  Subsystem5/2(cos(u)) -> Product1/2
  COG/1 -> Angle Conversion/1

== system AutopilotControlSystem/Navigation Filter/LLA to Flat Earth ==
  latLon : Inport
  h : Inport  Port=2
  COG : Inport  Port=3
  SOG : Inport  Port=4
  initPos : Inport  Port=5
  Enable : EnablePort
  LLA to Flat Earth : aerolibtransform2/LLA to Flat Earth  Commented=on  units=Metric (MKS)  ptype=Earth (WGS84)  F=1/298.257223563  R=6378137  LL0=[0 10]  psi=0
      settings: SourceProductName=Aerospace Blockset  SourceProductBaseCode=AE
  LLA to Flat Earth with Init Pos : mbdriLib/Coordinates/LLA to Flat Earth with Init Pos  R=6378137  F=1/298.2572235  psi=0
      settings: SourceProductName=Robotics System Toolbox  SourceProductBaseCode=RO
  Selector : Selector  InputPortWidth=3  IndexOptions=Index vector (dialog)  Indices=[3]  OutputSizes=1
  Selector1 : Selector  InputPortWidth=3  IndexOptions=Index vector (dialog)  Indices=[1 2]  OutputSizes=1
  Xe : Outport  VectorParamsAs1DForOutWhenUnconnected=off
  COG_out : Outport  Port=2  VectorParamsAs1DForOutWhenUnconnected=off
  SOG_out : Outport  Port=3  VectorParamsAs1DForOutWhenUnconnected=off
  wires:
  Selector1/1 -> LLA to Flat Earth with Init Pos/4
  SOG/1 -> SOG_out/1
  COG/1 -> COG_out/1
  Selector/1 -> LLA to Flat Earth with Init Pos/3
  latLon/1 -> LLA to Flat Earth with Init Pos/1
  initPos/1 -> Selector1/1, Selector/1
  h/1 -> LLA to Flat Earth with Init Pos/2
  LLA to Flat Earth with Init Pos/1 -> Xe/1

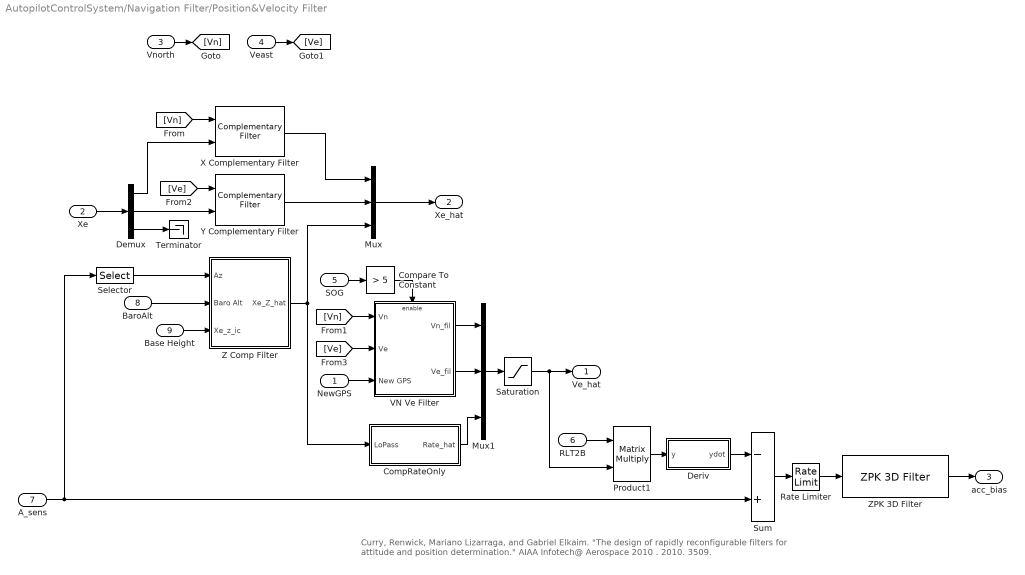
== system AutopilotControlSystem/Navigation Filter/Position&Velocity Filter ==
  note: Curry, Renwick, Mariano Lizarraga, and Gabriel Elkaim. "The design of rapidly reconfigurable filters for attitude and position determination." AIAA Infotech@ Aerospace 2010 . 2010. 3509.
  NewGPS : Inport
  Xe : Inport  Port=2
  Vnorth : Inport  Port=3
  Veast : Inport  Port=4
  SOG : Inport  Port=5
  RLT2B : Inport  Port=6
  A_sens : Inport  Port=7  Unit=m/s^2
  BaroAlt : Inport  Port=8
  Base Height : Inport  Port=9
  CompRateOnly : Subsystem  mask{omega=ap.cf.vzCutoff, T=ap.apSampleTime}
      mask prompts: omega "Cutoff Freq (rad/sec)"; T "Sample Time"
  Compare To Constant : simulink/Logic and Bit Operations/Compare To Constant  relop=>  const=5  OutDataTypeStr=boolean  ZeroCross=off
  Demux : Demux  Outputs=3
  "Deriv " : Subsystem
  Mux : Mux  Inputs=3
  Mux1 : Mux  Inputs=3
  Product1 : Product  Multiplication=Matrix(*)  RndMeth=Zero
  Rate Limiter : RateLimiter  RisingSlewLimit=ap.cf.accBiasRateLimit  FallingSlewLimit=-ap.cf.accBiasRateLimit  SampleTimeMode=inherited
  Saturation : Saturate  UpperLimit=40  LowerLimit=-40
      settings: AttributesFormatString="[%<LowerLimit>  %<UpperLimit>]"
  Selector : Selector  InputPortWidth=3  IndexOptions=Index vector (dialog)  Indices=[3]  OutputSizes=1
  Sum : Sum  Inputs=-+  OutDataTypeStr=single
  Terminator : Terminator
  VN Ve Filter : Subsystem
  X Complementary Filter : mbdriLib/Filtering/Complementary Filter  omega=ap.cf.xCutoff  T=ap.apSampleTime
      settings: SourceProductName=Robotics System Toolbox  SourceProductBaseCode=RO
  Y Complementary Filter : mbdriLib/Filtering/Complementary Filter  omega=ap.cf.yCutoff  T=ap.apSampleTime
      settings: SourceProductName=Robotics System Toolbox  SourceProductBaseCode=RO
  Z Comp Filter : Subsystem
  ZPK 3D Filter : mbdriLib/Filtering/ZPK 3D Filter  zval=[]  pval=-1/ap.cf.accBiasRateLimit  kval=1  TSample=ap.apSampleTime
      settings: SourceProductName=Robotics System Toolbox  SourceProductBaseCode=RO
  Ve_hat : Outport  VectorParamsAs1DForOutWhenUnconnected=off
  Xe_hat : Outport  Port=2  VectorParamsAs1DForOutWhenUnconnected=off
  acc_bias : Outport  Port=3  Unit=m/s^2  VectorParamsAs1DForOutWhenUnconnected=off
  wires:
  Saturation/1 -> Ve_hat/1, Product1/2
  Z Comp Filter/1(Xe_Z_hat) -> Mux/3, CompRateOnly/1(LoPass)
  BaroAlt/1 -> Z Comp Filter/2(Baro Alt)
  Demux/3 -> Terminator/1
  Selector/1 -> Z Comp Filter/1(Az)
  [Ve] -> VN Ve Filter/2(Ve)
  [Ve] -> Y Complementary Filter/1
  Veast/1 -> [Ve]
  [Vn] -> VN Ve Filter/1(Vn)
  [Vn] -> X Complementary Filter/1
  Vnorth/1 -> [Vn]
  CompRateOnly/1(Rate_hat) -> Mux1/3
  VN Ve Filter/2(Ve_fil) -> Mux1/2
  VN Ve Filter/1(Vn_fil) -> Mux1/1
  Mux/1 -> Xe_hat/1
  X Complementary Filter/1 -> Mux/1
  Y Complementary Filter/1 -> Mux/2
  Demux/2 -> Y Complementary Filter/2
  Demux/1 -> X Complementary Filter/2
  Xe/1 -> Demux/1
  Mux1/1 -> Saturation/1
  NewGPS/1 -> VN Ve Filter/3(New GPS)
  Compare To Constant/1 -> VN Ve Filter/Enable
  SOG/1 -> Compare To Constant/1
  Rate Limiter/1 -> ZPK 3D Filter/1
  ZPK 3D Filter/1 -> acc_bias/1
  Sum/1 -> Rate Limiter/1
  Product1/1 -> "Deriv "/1(y)
  "Deriv "/1(ydot) -> Sum/1
  A_sens/1 -> Selector/1, Sum/2
  RLT2B/1 -> Product1/1
  Base Height/1 -> Z Comp Filter/3(Xe_z_ic)

== system AutopilotControlSystem/SensorConditioning/Temperature Compensation ==
  Euler_raw : Inport
  Ab_raw : Inport  Port=2
  G_raw : Inport  Port=3
  q_raw : Inport  Port=4
  static_raw : Inport  Port=5
  T_raw : Inport  Port=6
  Euler_comp : Outport  VectorParamsAs1DForOutWhenUnconnected=off
  Ab_comp : Outport  Port=2  VectorParamsAs1DForOutWhenUnconnected=off
  G_comp : Outport  Port=3  VectorParamsAs1DForOutWhenUnconnected=off
  q_comp : Outport  Port=4  VectorParamsAs1DForOutWhenUnconnected=off
  static_comp : Outport  Port=5  VectorParamsAs1DForOutWhenUnconnected=off
  T_comp : Outport  Port=6  VectorParamsAs1DForOutWhenUnconnected=off
  wires:
  Euler_raw/1 -> Euler_comp/1
  Ab_raw/1 -> Ab_comp/1
  G_raw/1 -> G_comp/1
  q_raw/1 -> q_comp/1
  static_raw/1 -> static_comp/1
  T_raw/1 -> T_comp/1

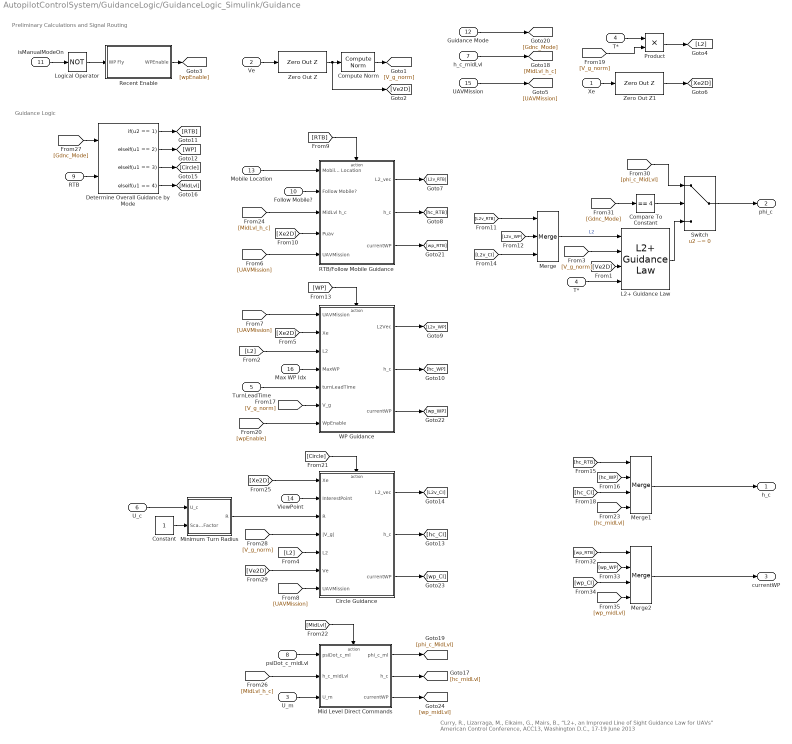
== system AutopilotControlSystem/GuidanceLogic/GuidanceLogic_Simulink/Guidance ==
  note: Curry, R., Lizarraga, M., Elkaim, G., Mairs, B., “L2+, an Improved Line of Sight Guidance Law for UAVs”
      | American Control Conference, ACC13, Washington D.C., 17-19 June 2013
  note: Preliminary Calculations and Signal Routing
  note: Guidance Logic
  Xe : Inport
  Ve : Inport  Port=2
  U_m : Inport  Port=3
  "T* " : Inport  Port=4
  TurnLeadTime : Inport  Port=5
  U_c : Inport  Port=6
  h_c_midLvl : Inport  Port=7
  psiDot_c_midLvl : Inport  Port=8
  RTB : Inport  Port=9
  Follow Mobile? : Inport  Port=10
  isManualModeOn : Inport  Port=11
  Guidance Mode : Inport  Port=12
  Mobile Location : Inport  Port=13
  ViewPoint : Inport  Port=14
  UAVMission : Inport  Port=15
  Max WP Idx : Inport  Port=16
  " Compute Norm" : mbdriLib/Utilities/ Compute Norm  SystemSampleTime=-1
      settings: SourceProductName=Robotics System Toolbox  SourceProductBaseCode=RO
  Circle Guidance : Subsystem  TreatAsAtomicUnit=on
  Compare To Constant : simulink/Logic and Bit Operations/Compare To Constant  relop===  const=4  OutDataTypeStr=boolean
  Constant : Constant  OutDataTypeStr=single
      settings: AttributesFormatString=%<Value>
  Determine Overall Guidance by Mode : If  NumInputs=2  IfExpression=u2 == 1  ElseIfExpressions=u1 == 2, u1 == 3, u1 == 4  ShowElse=off
  L2+ Guidance Law : mbdriLib/Guidance/L2+ Guidance Law  SystemSampleTime=-1
      settings: SourceProductName=Robotics System Toolbox  SourceProductBaseCode=RO
  Logical Operator : Logic  Operator=NOT  AllPortsSameDT=off  OutDataTypeStr=boolean
  Merge : Merge  Inputs=3  InitialOutput=[0 0 0]
  Merge1 : Merge  Inputs=4  InitialOutput=0
  Merge2 : Merge  Inputs=4  InitialOutput=0
  Mid Level Direct Commands : Subsystem  TreatAsAtomicUnit=on
  Minimum Turn Radius : Subsystem
  Product : Product
  RTB/Follow Mobile Guidance : Subsystem
  Recent Enable : Subsystem
  Switch : Switch  Criteria=u2 ~= 0  Threshold=3.1
  T* : InportShadow  Port=4
  WP Guidance : Subsystem  TreatAsAtomicUnit=on
  Zero Out Z : mbdriLib/Utilities/Zero Out Z  SystemSampleTime=-1
      settings: SourceProductName=Robotics System Toolbox  SourceProductBaseCode=RO
  Zero Out Z1 : mbdriLib/Utilities/Zero Out Z  SystemSampleTime=-1
      settings: SourceProductName=Robotics System Toolbox  SourceProductBaseCode=RO
  h_c : Outport  VectorParamsAs1DForOutWhenUnconnected=off
  phi_c : Outport  Port=2  Unit=rad  VectorParamsAs1DForOutWhenUnconnected=off
  currentWP : Outport  Port=3  VectorParamsAs1DForOutWhenUnconnected=off
  wires:
  [wp_midLvl] -> Merge2/4
  [wp_CI] -> Merge2/3
  [wp_WP] -> Merge2/2
  [wp_RTB] -> Merge2/1
  Merge2/1 -> currentWP/1
  Mid Level Direct Commands/3(currentWP) -> [wp_midLvl]
  Circle Guidance/3(currentWP) -> [wp_CI]
  WP Guidance/3(currentWP) -> [wp_WP]
  RTB/Follow Mobile Guidance/3(currentWP) -> [wp_RTB]
  U_m/1 -> Mid Level Direct Commands/3(U_m)
  [Gdnc_Mode] -> Compare To Constant/1
  [phi_c_MidLvl] -> Switch/1
  L2+ Guidance Law/1 -> Switch/3
  Switch/1 -> phi_c/1
  [Gdnc_Mode] -> Determine Overall Guidance by Mode/1
  Guidance Mode/1 -> [Gdnc_Mode]
  Mid Level Direct Commands/1(phi_c_ml) -> [phi_c_MidLvl]
  psiDot_c_midLvl/1 -> Mid Level Direct Commands/1(psiDot_c_ml)
  [MidLvl_h_c] -> Mid Level Direct Commands/2(h_c_midLvl)
  [MidLvl_h_c] -> RTB/Follow Mobile Guidance/3(MidLvl h_c)
  h_c_midLvl/1 -> [MidLvl_h_c]
  [hc_midLvl] -> Merge1/4
  Mid Level Direct Commands/2(h_c) -> [hc_midLvl]
  [MidLvl] -> Mid Level Direct Commands/Action
  [Circle] -> Circle Guidance/Action
  Determine Overall Guidance by Mode/4 -> [MidLvl]
  Determine Overall Guidance by Mode/3 -> [Circle]
  [WP] -> WP Guidance/Action
  Determine Overall Guidance by Mode/2 -> [WP]
  [RTB] -> RTB/Follow Mobile Guidance/Action
  Determine Overall Guidance by Mode/1 -> [RTB]
  [UAVMission] -> Circle Guidance/7(UAVMission)
  [UAVMission] -> WP Guidance/1(UAVMission)
  [UAVMission] -> RTB/Follow Mobile Guidance/5(UAVMission)
  UAVMission/1 -> [UAVMission]
  [L2] -> Circle Guidance/5(L2)
  Minimum Turn Radius/1(R) -> Circle Guidance/3(R)
  Max WP Idx/1 -> WP Guidance/4(MaxWP)
  [L2] -> WP Guidance/3(L2)
  Product/1 -> [L2]
  [Xe2D] -> WP Guidance/2(Xe)
  [wpEnable] -> WP Guidance/7(WpEnable)
  [V_g_norm] -> Product/2
  T*/1 -> Product/1
  TurnLeadTime/1 -> WP Guidance/5(turnLeadTime)
  [V_g_norm] -> WP Guidance/6(V_g)
  [hc_CI] -> Merge1/3
  Circle Guidance/2(h_c) -> [hc_CI]
  Circle Guidance/1(L2_vec) -> [L2v_CI]
  [Ve2D] -> Circle Guidance/6(Ve)
  [V_g_norm] -> Circle Guidance/4(|V_g|)
  Constant/1 -> Minimum Turn Radius/2(Scale Factor)
  U_c/1 -> Minimum Turn Radius/1(U_c)
  ViewPoint/1 -> Circle Guidance/2(InterestPoint)
  [Xe2D] -> Circle Guidance/1(Xe)
  Logical Operator/1 -> Recent Enable/1(WP Fly)
  isManualModeOn/1 -> Logical Operator/1
  [hc_WP] -> Merge1/2
  [hc_RTB] -> Merge1/1
  [L2v_CI] -> Merge/3
  [L2v_WP] -> Merge/2
  [L2v_RTB] -> Merge/1
  WP Guidance/2(h_c) -> [hc_WP]
  WP Guidance/1(L2Vec) -> [L2v_WP]
  RTB/Follow Mobile Guidance/2(h_c) -> [hc_RTB]
  RTB/Follow Mobile Guidance/1(L2_vec) -> [L2v_RTB]
  Merge1/1 -> h_c/1
  [Xe2D] -> RTB/Follow Mobile Guidance/4(Puav)
  Zero Out Z1/1 -> [Xe2D]
  Xe/1 -> Zero Out Z1/1
  Zero Out Z/1 -> [Ve2D], " Compute Norm"/1
  Mobile Location/1 -> RTB/Follow Mobile Guidance/1(Mobile Location)
  Follow Mobile?/1 -> RTB/Follow Mobile Guidance/2(Follow Mobile?)
  RTB/1 -> Determine Overall Guidance by Mode/2
  Recent Enable/1(WPEnable) -> [wpEnable]
  "T* "/1 -> L2+ Guidance Law/4
  " Compute Norm"/1 -> [V_g_norm]
  Ve/1 -> Zero Out Z/1
  Compare To Constant/1 -> Switch/2
  Merge/1 -> L2+ Guidance Law/1  "L2"
  [V_g_norm] -> L2+ Guidance Law/2
  [Ve2D] -> L2+ Guidance Law/3

== system AutopilotControlSystem/GuidanceLogic/GuidanceLogic_Stateflow/GuidanceStateMachine/GuidanceLogic.MidLevel ==
  gsCommands : Inport
  U_m : Inport  Port=2
  " " : ActionPort
      settings: CopyFcn=Stateflow.SLINSF.SimulinkMan.removeBlockPreDeleteFcn  PreDeleteFcn=Stateflow.SLINSF.SimulinkMan.unsafePredeleteFcn
  Bus Selector : BusSelector  OutputSignals=psiDot_c_midLevel,h_c_midLevel
  RTB1 : Constant  Value=0  OutDataTypeStr=uint8
      settings: AttributesFormatString=%<Value>
  psi_dot to phi : mbdriLib/Angles and Units/psi_dot to phi  SystemSampleTime=-1  Latency=0  AutoFrameSizeCalculation=off
      settings: SourceProductName=Robotics System Toolbox  SourceProductBaseCode=RO
  currentWP : Outport  VectorParamsAs1DForOutWhenUnconnected=off
  h_c : Outport  Port=2  VectorParamsAs1DForOutWhenUnconnected=off
  phi_c_ml : Outport  Port=3  VectorParamsAs1DForOutWhenUnconnected=off
  wires:
  Bus Selector/2 -> h_c/1  "<h_c_midLevel>"
  RTB1/1 -> currentWP/1
  Bus Selector/1 -> psi_dot to phi/1  "<psiDot_c_midLevel>"
  psi_dot to phi/1 -> phi_c_ml/1
  U_m/1 -> psi_dot to phi/2
  gsCommands/1 -> Bus Selector/1
